simulink model "statelessWriter2_2"  (Simulink 8.8)
settings: Solver=VariableStepAuto  StartTime=0.0  StopTime=10.0  RelTol=1e-3
settings Model: SuppressorTable=22 serialization::archive 11 0 3 0 0 0 11 0  Creator=root  LastModifiedBy=root
settings DataIOCC: LimitDataPoints=off  SaveFormat=Dataset  SignalLoggingSaveFormat=Dataset
settings OptimizationCC: LifeSpan=auto
settings DebuggingCC: UnderspecifiedInitializationDetection=Simplified  MergeDetectMultiDrivingBlocksExec=error  FcnCallInpInsideContextMsg=error  StateNameClashWarn=none  SFUnexpectedBacktrackingDiag=error  SFNoUnconditionalDefaultTransitionDiag=error  SFExecutionAtInitializationDiag=warning
settings HardwareCC: ProdBitPerPointer=64  ProdBitPerSizeT=64  ProdBitPerPtrDiffT=64  ProdLargestAtomicFloat=Float  ProdIntDivRoundTo=Zero  ProdEndianess=LittleEndian  ProdWordSize=64  ProdHWDeviceType=Intel->x86-64 (Windows64)
settings ModelReferenceCC: PropagateSignalLabelsOutOfModel=on
settings GRTTargetCC: TargetLangStandard=C99 (ISO)  GeneratePreprocessorConditionals=Use local settings  CombineOutputUpdateFcns=on  GRTInterface=off
settings ConfigComp: CovMetricSettings=dwe  CovHtmlReporting=off  CovSaveCumulativeToWorkspaceVar=off  CovSaveSingleToWorkspaceVar=off  CovExternalEMLEnable=on

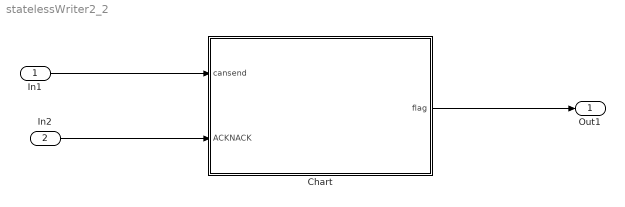
== system statelessWriter2_2 ==
  In1 : Inport
  In2 : Inport  Port=2
  Chart : Stateflow chart  TreatAsAtomicUnit=on
  Out1 : Outport
  wires:
  In1/1 -> Chart/1(cansend)
  In2/1 -> Chart/2(ACKNACK)
  Chart/1(flag) -> Out1/1

== stateflow chart Chart ==
  state repairing
    during:flag=0
  state waiting
    during:flag=1;
  state must_repair
    during:flag=1;
  repairing -> repairing [order 1] : [cansend]/{re_changes = re_changes - 1}
  must_repair -> repairing [order 1] : after(ResponseDelay,sec)
  must_repair -> must_repair [order 2] : [ACKNACK]/{re_changes = re_changes + 1}
  repairing -> waiting [order 2] : [re_changes==0]
  waiting -> must_repair [order 2] : [re_changes>0]
  (default) -> waiting : {re_changes=0}
  waiting -> waiting [order 1] : [ACKNACK]/{re_changes = re_changes + 1}
  data: flag output double; cansend input double; re_changes local double; ACKNACK input double; ResponseDelay constant double
  events: event local FUNCTION_CALL_EVENT; event1 local FUNCTION_CALL_EVENT
